simulink model "Lab2_P1B1"  (R2025b)
settings: Solver=VariableStepAuto  StartTime=0.0  StopTime=2.0  RelTol=1e-3
settings Model: Creator=safiakhalil  LastModifiedBy=safiakhalil

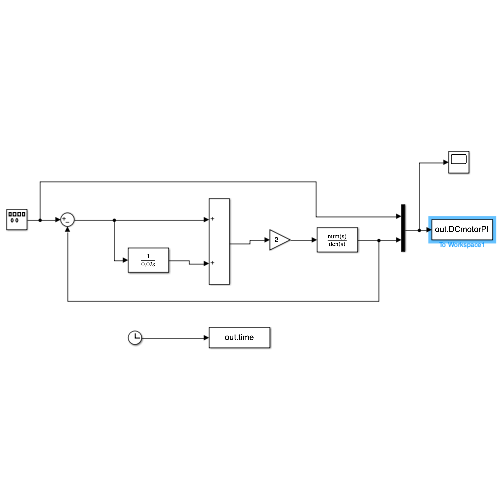
[thumbnail: Simulink's stored preview of the top-level diagram]
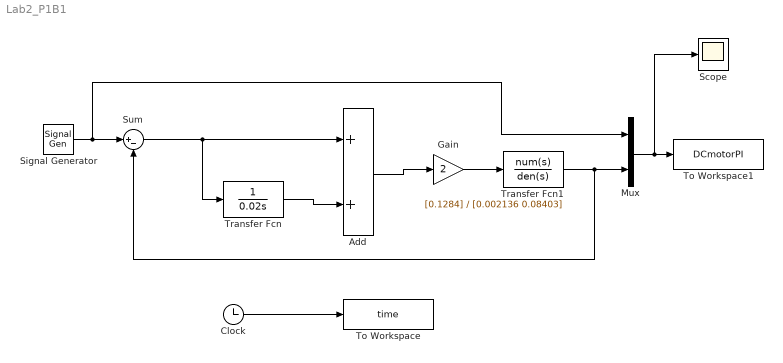
== system Lab2_P1B1 ==
  Add : Sum
  Clock : Clock
  Gain : Gain  Gain=2
  Mux : Mux  Inputs=2
  Scope : Scope
      settings: ActiveDisplayYMinimum=-1  ActiveDisplayYMaximum=1
  Signal Generator : SignalGenerator  WaveForm=square  Amplitude=1.5  Frequency=2
  Sum : Sum  Inputs=|+-
  To Workspace : ToWorkspace  VariableName=time  SampleTime=-1
  To Workspace1 : ToWorkspace  VariableName=DCmotorPI  SampleTime=-1
  Transfer Fcn : TransferFcn  Denominator=[0.02 0]
  Transfer Fcn1 : TransferFcn  Numerator=[0.1284]  Denominator=[0.002136 0.08403]
  wires:
  Transfer Fcn/1 -> Add/2
  Sum/1 -> Transfer Fcn/1, Add/1
  Signal Generator/1 -> Mux/1, Sum/1
  Add/1 -> Gain/1
  Clock/1 -> To Workspace/1
  Mux/1 -> Scope/1, To Workspace1/1
  Gain/1 -> Transfer Fcn1/1
  Transfer Fcn1/1 -> Sum/2, Mux/2
